simulink model "SCex4_3"  (R2024b)
settings: Solver=VariableStepAuto  StartTime=0.0  StopTime=10.0  RelTol=1e-3
libraries: simulink x2
settings Model: Creator=pedro  LastModifiedBy=pedro

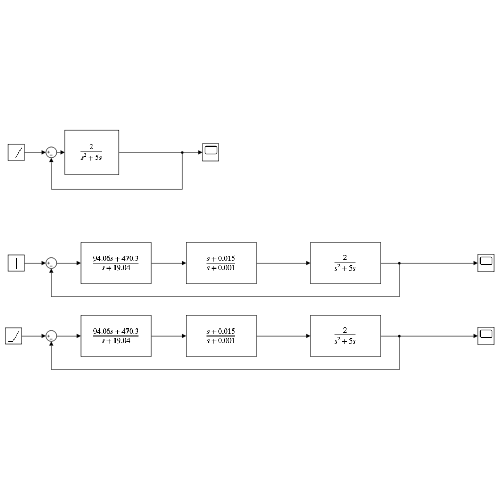
[thumbnail: Simulink's stored preview of the top-level diagram]
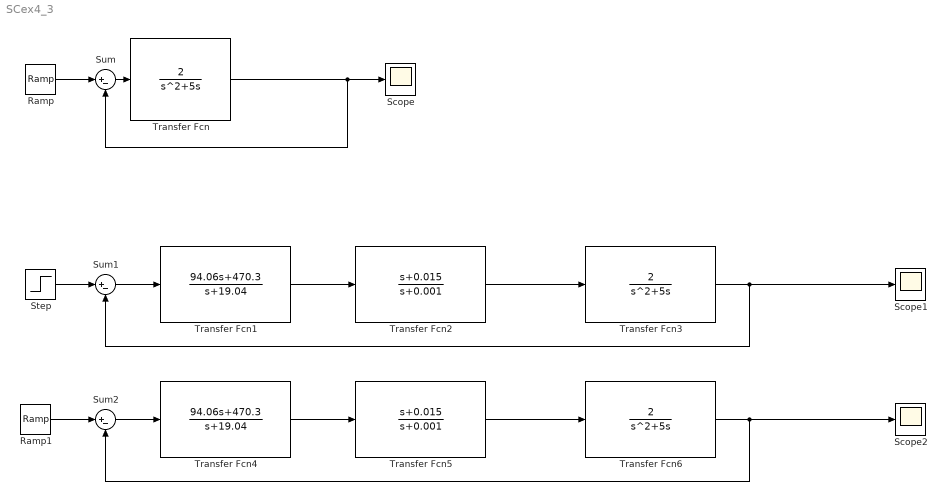
== system SCex4_3 ==
  Ramp : simulink/Sources/Ramp  slope=1  start=0  InitialOutput=0
  Ramp1 : simulink/Sources/Ramp  slope=1  start=0  InitialOutput=0
  Scope : Scope
  Scope1 : Scope
  Scope2 : Scope
  Step : Step  SampleTime=0
  Sum : Sum  Inputs=|+-
  Sum1 : Sum  Inputs=|+-
  Sum2 : Sum  Inputs=|+-
  Transfer Fcn : TransferFcn  Numerator=[2]  Denominator=[1 5 0]
  Transfer Fcn1 : TransferFcn  Numerator=[94.06 470.3]  Denominator=[1 19.04]
  Transfer Fcn2 : TransferFcn  Numerator=[1 0.015]  Denominator=[1 0.001]
  Transfer Fcn3 : TransferFcn  Numerator=[2]  Denominator=[1 5 0]
  Transfer Fcn4 : TransferFcn  Numerator=[94.06 470.3]  Denominator=[1 19.04]
  Transfer Fcn5 : TransferFcn  Numerator=[1 0.015]  Denominator=[1 0.001]
  Transfer Fcn6 : TransferFcn  Numerator=[2]  Denominator=[1 5 0]
  wires:
  Transfer Fcn/1 -> Sum/2, Scope/1
  Sum/1 -> Transfer Fcn/1
  Ramp/1 -> Sum/1
  Sum1/1 -> Transfer Fcn1/1
  Step/1 -> Sum1/1
  Transfer Fcn1/1 -> Transfer Fcn2/1
  Transfer Fcn2/1 -> Transfer Fcn3/1
  Transfer Fcn3/1 -> Sum1/2, Scope1/1
  Transfer Fcn4/1 -> Transfer Fcn5/1
  Ramp1/1 -> Sum2/1
  Transfer Fcn6/1 -> Sum2/2, Scope2/1
  Transfer Fcn5/1 -> Transfer Fcn6/1
  Sum2/1 -> Transfer Fcn4/1
